simulink model "bit32cpu"  (R2020a)
settings: Solver=VariableStepAuto  StartTime=0.0  StopTime=10.0  RelTol=1e-3
libraries: simulink_extras x392
(part 17 of 63)

== system bit32cpu/ALU/Subsystem7/Subsystem3/Subsystem4/Subsystem5 ==
  In1 : Inport
  In2 : Inport  Port=2
  In3 : Inport  Port=3
  In4 : Inport  Port=4
  In5 : Inport  Port=5
  In6 : Inport  Port=6
  In7 : Inport  Port=7
  NAND : Logic  Operator=NAND  AllPortsSameDT=off  OutDataTypeStr=boolean
  NAND{1..2,4..6} (5 alike) : Logic  Operator=NAND  Inputs=4  AllPortsSameDT=off  OutDataTypeStr=boolean
  NAND3 : Logic  Operator=NAND  AllPortsSameDT=off  OutDataTypeStr=boolean
  Out1 : Outport
  wires:
  NAND6/1 -> NAND1/4
  In5/1 -> NAND5/3
  NAND3/1 -> NAND4/2, NAND2/2
  In1/1 -> NAND6/2, NAND5/2, NAND3/2, NAND3/1
  In2/1 -> NAND6/1, NAND4/1, NAND/2, NAND/1
  In4/1 -> NAND4/3
  In3/1 -> NAND2/3
  NAND/1 -> NAND5/1, NAND2/1
  NAND1/1 -> Out1/1
  In6/1 -> NAND6/3
  NAND5/1 -> NAND1/3
  NAND4/1 -> NAND1/2
  In7/1 -> NAND2/4, NAND4/4, NAND5/4, NAND6/4
  NAND2/1 -> NAND1/1

== system bit32cpu/ALU/Subsystem7/Subsystem3/Subsystem4/Subsystem6 ==
  In1 : Inport
  In2 : Inport  Port=2
  In3 : Inport  Port=3
  In4 : Inport  Port=4
  In5 : Inport  Port=5
  In6 : Inport  Port=6
  In7 : Inport  Port=7
  NAND : Logic  Operator=NAND  AllPortsSameDT=off  OutDataTypeStr=boolean
  NAND{1..2,4..6} (5 alike) : Logic  Operator=NAND  Inputs=4  AllPortsSameDT=off  OutDataTypeStr=boolean
  NAND3 : Logic  Operator=NAND  AllPortsSameDT=off  OutDataTypeStr=boolean
  Out1 : Outport
  wires:
  NAND6/1 -> NAND1/4
  In5/1 -> NAND5/3
  NAND3/1 -> NAND4/2, NAND2/2
  In1/1 -> NAND6/2, NAND5/2, NAND3/2, NAND3/1
  In2/1 -> NAND6/1, NAND4/1, NAND/2, NAND/1
  In4/1 -> NAND4/3
  In3/1 -> NAND2/3
  NAND/1 -> NAND5/1, NAND2/1
  NAND1/1 -> Out1/1
  In6/1 -> NAND6/3
  NAND5/1 -> NAND1/3
  NAND4/1 -> NAND1/2
  In7/1 -> NAND2/4, NAND4/4, NAND5/4, NAND6/4
  NAND2/1 -> NAND1/1

== system bit32cpu/ALU/Subsystem7/Subsystem3/Subsystem4/Subsystem7 ==
  In1 : Inport
  In2 : Inport  Port=2
  In3 : Inport  Port=3
  In4 : Inport  Port=4
  In5 : Inport  Port=5
  In6 : Inport  Port=6
  In7 : Inport  Port=7
  NAND : Logic  Operator=NAND  AllPortsSameDT=off  OutDataTypeStr=boolean
  NAND{1..2,4..6} (5 alike) : Logic  Operator=NAND  Inputs=4  AllPortsSameDT=off  OutDataTypeStr=boolean
  NAND3 : Logic  Operator=NAND  AllPortsSameDT=off  OutDataTypeStr=boolean
  Out1 : Outport
  wires:
  NAND6/1 -> NAND1/4
  In5/1 -> NAND5/3
  NAND3/1 -> NAND4/2, NAND2/2
  In1/1 -> NAND6/2, NAND5/2, NAND3/2, NAND3/1
  In2/1 -> NAND6/1, NAND4/1, NAND/2, NAND/1
  In4/1 -> NAND4/3
  In3/1 -> NAND2/3
  NAND/1 -> NAND5/1, NAND2/1
  NAND1/1 -> Out1/1
  In6/1 -> NAND6/3
  NAND5/1 -> NAND1/3
  NAND4/1 -> NAND1/2
  In7/1 -> NAND2/4, NAND4/4, NAND5/4, NAND6/4
  NAND2/1 -> NAND1/1

== system bit32cpu/ALU/Subsystem7/Subsystem3/Subsystem5/Subsystem ==
  In1 : Inport
  In2 : Inport  Port=2
  In3 : Inport  Port=3
  In4 : Inport  Port=4
  In5 : Inport  Port=5
  In6 : Inport  Port=6
  In7 : Inport  Port=7
  NAND : Logic  Operator=NAND  AllPortsSameDT=off  OutDataTypeStr=boolean
  NAND{1..2,4..6} (5 alike) : Logic  Operator=NAND  Inputs=4  AllPortsSameDT=off  OutDataTypeStr=boolean
  NAND3 : Logic  Operator=NAND  AllPortsSameDT=off  OutDataTypeStr=boolean
  Out1 : Outport
  wires:
  NAND6/1 -> NAND1/4
  In5/1 -> NAND5/3
  NAND3/1 -> NAND4/2, NAND2/2
  In1/1 -> NAND6/2, NAND5/2, NAND3/2, NAND3/1
  In2/1 -> NAND6/1, NAND4/1, NAND/2, NAND/1
  In4/1 -> NAND4/3
  In3/1 -> NAND2/3
  NAND/1 -> NAND5/1, NAND2/1
  NAND1/1 -> Out1/1
  In6/1 -> NAND6/3
  NAND5/1 -> NAND1/3
  NAND4/1 -> NAND1/2
  In7/1 -> NAND2/4, NAND4/4, NAND5/4, NAND6/4
  NAND2/1 -> NAND1/1

== system bit32cpu/ALU/Subsystem7/Subsystem3/Subsystem5/Subsystem1 ==
  In1 : Inport
  In2 : Inport  Port=2
  In3 : Inport  Port=3
  In4 : Inport  Port=4
  In5 : Inport  Port=5
  In6 : Inport  Port=6
  In7 : Inport  Port=7
  NAND : Logic  Operator=NAND  AllPortsSameDT=off  OutDataTypeStr=boolean
  NAND{1..2,4..6} (5 alike) : Logic  Operator=NAND  Inputs=4  AllPortsSameDT=off  OutDataTypeStr=boolean
  NAND3 : Logic  Operator=NAND  AllPortsSameDT=off  OutDataTypeStr=boolean
  Out1 : Outport
  wires:
  NAND6/1 -> NAND1/4
  In5/1 -> NAND5/3
  NAND3/1 -> NAND4/2, NAND2/2
  In1/1 -> NAND6/2, NAND5/2, NAND3/2, NAND3/1
  In2/1 -> NAND6/1, NAND4/1, NAND/2, NAND/1
  In4/1 -> NAND4/3
  In3/1 -> NAND2/3
  NAND/1 -> NAND5/1, NAND2/1
  NAND1/1 -> Out1/1
  In6/1 -> NAND6/3
  NAND5/1 -> NAND1/3
  NAND4/1 -> NAND1/2
  In7/1 -> NAND2/4, NAND4/4, NAND5/4, NAND6/4
  NAND2/1 -> NAND1/1

== system bit32cpu/ALU/Subsystem7/Subsystem3/Subsystem5/Subsystem2 ==
  In1 : Inport
  In2 : Inport  Port=2
  In3 : Inport  Port=3
  In4 : Inport  Port=4
  In5 : Inport  Port=5
  In6 : Inport  Port=6
  In7 : Inport  Port=7
  NAND : Logic  Operator=NAND  AllPortsSameDT=off  OutDataTypeStr=boolean
  NAND{1..2,4..6} (5 alike) : Logic  Operator=NAND  Inputs=4  AllPortsSameDT=off  OutDataTypeStr=boolean
  NAND3 : Logic  Operator=NAND  AllPortsSameDT=off  OutDataTypeStr=boolean
  Out1 : Outport
  wires:
  NAND6/1 -> NAND1/4
  In5/1 -> NAND5/3
  NAND3/1 -> NAND4/2, NAND2/2
  In1/1 -> NAND6/2, NAND5/2, NAND3/2, NAND3/1
  In2/1 -> NAND6/1, NAND4/1, NAND/2, NAND/1
  In4/1 -> NAND4/3
  In3/1 -> NAND2/3
  NAND/1 -> NAND5/1, NAND2/1
  NAND1/1 -> Out1/1
  In6/1 -> NAND6/3
  NAND5/1 -> NAND1/3
  NAND4/1 -> NAND1/2
  In7/1 -> NAND2/4, NAND4/4, NAND5/4, NAND6/4
  NAND2/1 -> NAND1/1

== system bit32cpu/ALU/Subsystem7/Subsystem3/Subsystem5/Subsystem3 ==
  In1 : Inport
  In2 : Inport  Port=2
  In3 : Inport  Port=3
  In4 : Inport  Port=4
  In5 : Inport  Port=5
  In6 : Inport  Port=6
  In7 : Inport  Port=7
  NAND : Logic  Operator=NAND  AllPortsSameDT=off  OutDataTypeStr=boolean
  NAND{1..2,4..6} (5 alike) : Logic  Operator=NAND  Inputs=4  AllPortsSameDT=off  OutDataTypeStr=boolean
  NAND3 : Logic  Operator=NAND  AllPortsSameDT=off  OutDataTypeStr=boolean
  Out1 : Outport
  wires:
  NAND6/1 -> NAND1/4
  In5/1 -> NAND5/3
  NAND3/1 -> NAND4/2, NAND2/2
  In1/1 -> NAND6/2, NAND5/2, NAND3/2, NAND3/1
  In2/1 -> NAND6/1, NAND4/1, NAND/2, NAND/1
  In4/1 -> NAND4/3
  In3/1 -> NAND2/3
  NAND/1 -> NAND5/1, NAND2/1
  NAND1/1 -> Out1/1
  In6/1 -> NAND6/3
  NAND5/1 -> NAND1/3
  NAND4/1 -> NAND1/2
  In7/1 -> NAND2/4, NAND4/4, NAND5/4, NAND6/4
  NAND2/1 -> NAND1/1

== system bit32cpu/ALU/Subsystem7/Subsystem3/Subsystem5/Subsystem4 ==
  In1 : Inport
  In2 : Inport  Port=2
  In3 : Inport  Port=3
  In4 : Inport  Port=4
  In5 : Inport  Port=5
  In6 : Inport  Port=6
  In7 : Inport  Port=7
  NAND : Logic  Operator=NAND  AllPortsSameDT=off  OutDataTypeStr=boolean
  NAND{1..2,4..6} (5 alike) : Logic  Operator=NAND  Inputs=4  AllPortsSameDT=off  OutDataTypeStr=boolean
  NAND3 : Logic  Operator=NAND  AllPortsSameDT=off  OutDataTypeStr=boolean
  Out1 : Outport
  wires:
  NAND6/1 -> NAND1/4
  In5/1 -> NAND5/3
  NAND3/1 -> NAND4/2, NAND2/2
  In1/1 -> NAND6/2, NAND5/2, NAND3/2, NAND3/1
  In2/1 -> NAND6/1, NAND4/1, NAND/2, NAND/1
  In4/1 -> NAND4/3
  In3/1 -> NAND2/3
  NAND/1 -> NAND5/1, NAND2/1
  NAND1/1 -> Out1/1
  In6/1 -> NAND6/3
  NAND5/1 -> NAND1/3
  NAND4/1 -> NAND1/2
  In7/1 -> NAND2/4, NAND4/4, NAND5/4, NAND6/4
  NAND2/1 -> NAND1/1

== system bit32cpu/ALU/Subsystem7/Subsystem3/Subsystem5/Subsystem5 ==
  In1 : Inport
  In2 : Inport  Port=2
  In3 : Inport  Port=3
  In4 : Inport  Port=4
  In5 : Inport  Port=5
  In6 : Inport  Port=6
  In7 : Inport  Port=7
  NAND : Logic  Operator=NAND  AllPortsSameDT=off  OutDataTypeStr=boolean
  NAND{1..2,4..6} (5 alike) : Logic  Operator=NAND  Inputs=4  AllPortsSameDT=off  OutDataTypeStr=boolean
  NAND3 : Logic  Operator=NAND  AllPortsSameDT=off  OutDataTypeStr=boolean
  Out1 : Outport
  wires:
  NAND6/1 -> NAND1/4
  In5/1 -> NAND5/3
  NAND3/1 -> NAND4/2, NAND2/2
  In1/1 -> NAND6/2, NAND5/2, NAND3/2, NAND3/1
  In2/1 -> NAND6/1, NAND4/1, NAND/2, NAND/1
  In4/1 -> NAND4/3
  In3/1 -> NAND2/3
  NAND/1 -> NAND5/1, NAND2/1
  NAND1/1 -> Out1/1
  In6/1 -> NAND6/3
  NAND5/1 -> NAND1/3
  NAND4/1 -> NAND1/2
  In7/1 -> NAND2/4, NAND4/4, NAND5/4, NAND6/4
  NAND2/1 -> NAND1/1

== system bit32cpu/ALU/Subsystem7/Subsystem3/Subsystem5/Subsystem6 ==
  In1 : Inport
  In2 : Inport  Port=2
  In3 : Inport  Port=3
  In4 : Inport  Port=4
  In5 : Inport  Port=5
  In6 : Inport  Port=6
  In7 : Inport  Port=7
  NAND : Logic  Operator=NAND  AllPortsSameDT=off  OutDataTypeStr=boolean
  NAND{1..2,4..6} (5 alike) : Logic  Operator=NAND  Inputs=4  AllPortsSameDT=off  OutDataTypeStr=boolean
  NAND3 : Logic  Operator=NAND  AllPortsSameDT=off  OutDataTypeStr=boolean
  Out1 : Outport
  wires:
  NAND6/1 -> NAND1/4
  In5/1 -> NAND5/3
  NAND3/1 -> NAND4/2, NAND2/2
  In1/1 -> NAND6/2, NAND5/2, NAND3/2, NAND3/1
  In2/1 -> NAND6/1, NAND4/1, NAND/2, NAND/1
  In4/1 -> NAND4/3
  In3/1 -> NAND2/3
  NAND/1 -> NAND5/1, NAND2/1
  NAND1/1 -> Out1/1
  In6/1 -> NAND6/3
  NAND5/1 -> NAND1/3
  NAND4/1 -> NAND1/2
  In7/1 -> NAND2/4, NAND4/4, NAND5/4, NAND6/4
  NAND2/1 -> NAND1/1

== system bit32cpu/ALU/Subsystem7/Subsystem3/Subsystem5/Subsystem7 ==
  In1 : Inport
  In2 : Inport  Port=2
  In3 : Inport  Port=3
  In4 : Inport  Port=4
  In5 : Inport  Port=5
  In6 : Inport  Port=6
  In7 : Inport  Port=7
  NAND : Logic  Operator=NAND  AllPortsSameDT=off  OutDataTypeStr=boolean
  NAND{1..2,4..6} (5 alike) : Logic  Operator=NAND  Inputs=4  AllPortsSameDT=off  OutDataTypeStr=boolean
  NAND3 : Logic  Operator=NAND  AllPortsSameDT=off  OutDataTypeStr=boolean
  Out1 : Outport
  wires:
  NAND6/1 -> NAND1/4
  In5/1 -> NAND5/3
  NAND3/1 -> NAND4/2, NAND2/2
  In1/1 -> NAND6/2, NAND5/2, NAND3/2, NAND3/1
  In2/1 -> NAND6/1, NAND4/1, NAND/2, NAND/1
  In4/1 -> NAND4/3
  In3/1 -> NAND2/3
  NAND/1 -> NAND5/1, NAND2/1
  NAND1/1 -> Out1/1
  In6/1 -> NAND6/3
  NAND5/1 -> NAND1/3
  NAND4/1 -> NAND1/2
  In7/1 -> NAND2/4, NAND4/4, NAND5/4, NAND6/4
  NAND2/1 -> NAND1/1

== system bit32cpu/ALU/Subsystem7/Subsystem4/Subsystem1/Subsystem ==
  In1 : Inport
  In2 : Inport  Port=2
  In3 : Inport  Port=3
  In4 : Inport  Port=4
  In5 : Inport  Port=5
  In6 : Inport  Port=6
  In7 : Inport  Port=7
  NAND : Logic  Operator=NAND  AllPortsSameDT=off  OutDataTypeStr=boolean
  NAND{1..2,4..6} (5 alike) : Logic  Operator=NAND  Inputs=4  AllPortsSameDT=off  OutDataTypeStr=boolean
  NAND3 : Logic  Operator=NAND  AllPortsSameDT=off  OutDataTypeStr=boolean
  Out1 : Outport
  wires:
  NAND6/1 -> NAND1/4
  In5/1 -> NAND5/3
  NAND3/1 -> NAND4/2, NAND2/2
  In1/1 -> NAND6/2, NAND5/2, NAND3/2, NAND3/1
  In2/1 -> NAND6/1, NAND4/1, NAND/2, NAND/1
  In4/1 -> NAND4/3
  In3/1 -> NAND2/3
  NAND/1 -> NAND5/1, NAND2/1
  NAND1/1 -> Out1/1
  In6/1 -> NAND6/3
  NAND5/1 -> NAND1/3
  NAND4/1 -> NAND1/2
  In7/1 -> NAND2/4, NAND4/4, NAND5/4, NAND6/4
  NAND2/1 -> NAND1/1

== system bit32cpu/ALU/Subsystem7/Subsystem4/Subsystem1/Subsystem1 ==
  In1 : Inport
  In2 : Inport  Port=2
  In3 : Inport  Port=3
  In4 : Inport  Port=4
  In5 : Inport  Port=5
  In6 : Inport  Port=6
  In7 : Inport  Port=7
  NAND : Logic  Operator=NAND  AllPortsSameDT=off  OutDataTypeStr=boolean
  NAND{1..2,4..6} (5 alike) : Logic  Operator=NAND  Inputs=4  AllPortsSameDT=off  OutDataTypeStr=boolean
  NAND3 : Logic  Operator=NAND  AllPortsSameDT=off  OutDataTypeStr=boolean
  Out1 : Outport
  wires:
  NAND6/1 -> NAND1/4
  In5/1 -> NAND5/3
  NAND3/1 -> NAND4/2, NAND2/2
  In1/1 -> NAND6/2, NAND5/2, NAND3/2, NAND3/1
  In2/1 -> NAND6/1, NAND4/1, NAND/2, NAND/1
  In4/1 -> NAND4/3
  In3/1 -> NAND2/3
  NAND/1 -> NAND5/1, NAND2/1
  NAND1/1 -> Out1/1
  In6/1 -> NAND6/3
  NAND5/1 -> NAND1/3
  NAND4/1 -> NAND1/2
  In7/1 -> NAND2/4, NAND4/4, NAND5/4, NAND6/4
  NAND2/1 -> NAND1/1

== system bit32cpu/ALU/Subsystem7/Subsystem4/Subsystem1/Subsystem2 ==
  In1 : Inport
  In2 : Inport  Port=2
  In3 : Inport  Port=3
  In4 : Inport  Port=4
  In5 : Inport  Port=5
  In6 : Inport  Port=6
  In7 : Inport  Port=7
  NAND : Logic  Operator=NAND  AllPortsSameDT=off  OutDataTypeStr=boolean
  NAND{1..2,4..6} (5 alike) : Logic  Operator=NAND  Inputs=4  AllPortsSameDT=off  OutDataTypeStr=boolean
  NAND3 : Logic  Operator=NAND  AllPortsSameDT=off  OutDataTypeStr=boolean
  Out1 : Outport
  wires:
  NAND6/1 -> NAND1/4
  In5/1 -> NAND5/3
  NAND3/1 -> NAND4/2, NAND2/2
  In1/1 -> NAND6/2, NAND5/2, NAND3/2, NAND3/1
  In2/1 -> NAND6/1, NAND4/1, NAND/2, NAND/1
  In4/1 -> NAND4/3
  In3/1 -> NAND2/3
  NAND/1 -> NAND5/1, NAND2/1
  NAND1/1 -> Out1/1
  In6/1 -> NAND6/3
  NAND5/1 -> NAND1/3
  NAND4/1 -> NAND1/2
  In7/1 -> NAND2/4, NAND4/4, NAND5/4, NAND6/4
  NAND2/1 -> NAND1/1

== system bit32cpu/ALU/Subsystem7/Subsystem4/Subsystem1/Subsystem3 ==
  In1 : Inport
  In2 : Inport  Port=2
  In3 : Inport  Port=3
  In4 : Inport  Port=4
  In5 : Inport  Port=5
  In6 : Inport  Port=6
  In7 : Inport  Port=7
  NAND : Logic  Operator=NAND  AllPortsSameDT=off  OutDataTypeStr=boolean
  NAND{1..2,4..6} (5 alike) : Logic  Operator=NAND  Inputs=4  AllPortsSameDT=off  OutDataTypeStr=boolean
  NAND3 : Logic  Operator=NAND  AllPortsSameDT=off  OutDataTypeStr=boolean
  Out1 : Outport
  wires:
  NAND6/1 -> NAND1/4
  In5/1 -> NAND5/3
  NAND3/1 -> NAND4/2, NAND2/2
  In1/1 -> NAND6/2, NAND5/2, NAND3/2, NAND3/1
  In2/1 -> NAND6/1, NAND4/1, NAND/2, NAND/1
  In4/1 -> NAND4/3
  In3/1 -> NAND2/3
  NAND/1 -> NAND5/1, NAND2/1
  NAND1/1 -> Out1/1
  In6/1 -> NAND6/3
  NAND5/1 -> NAND1/3
  NAND4/1 -> NAND1/2
  In7/1 -> NAND2/4, NAND4/4, NAND5/4, NAND6/4
  NAND2/1 -> NAND1/1

== system bit32cpu/ALU/Subsystem7/Subsystem4/Subsystem1/Subsystem4 ==
  In1 : Inport
  In2 : Inport  Port=2
  In3 : Inport  Port=3
  In4 : Inport  Port=4
  In5 : Inport  Port=5
  In6 : Inport  Port=6
  In7 : Inport  Port=7
  NAND : Logic  Operator=NAND  AllPortsSameDT=off  OutDataTypeStr=boolean
  NAND{1..2,4..6} (5 alike) : Logic  Operator=NAND  Inputs=4  AllPortsSameDT=off  OutDataTypeStr=boolean
  NAND3 : Logic  Operator=NAND  AllPortsSameDT=off  OutDataTypeStr=boolean
  Out1 : Outport
  wires:
  NAND6/1 -> NAND1/4
  In5/1 -> NAND5/3
  NAND3/1 -> NAND4/2, NAND2/2
  In1/1 -> NAND6/2, NAND5/2, NAND3/2, NAND3/1
  In2/1 -> NAND6/1, NAND4/1, NAND/2, NAND/1
  In4/1 -> NAND4/3
  In3/1 -> NAND2/3
  NAND/1 -> NAND5/1, NAND2/1
  NAND1/1 -> Out1/1
  In6/1 -> NAND6/3
  NAND5/1 -> NAND1/3
  NAND4/1 -> NAND1/2
  In7/1 -> NAND2/4, NAND4/4, NAND5/4, NAND6/4
  NAND2/1 -> NAND1/1

== system bit32cpu/ALU/Subsystem7/Subsystem4/Subsystem1/Subsystem5 ==
  In1 : Inport
  In2 : Inport  Port=2
  In3 : Inport  Port=3
  In4 : Inport  Port=4
  In5 : Inport  Port=5
  In6 : Inport  Port=6
  In7 : Inport  Port=7
  NAND : Logic  Operator=NAND  AllPortsSameDT=off  OutDataTypeStr=boolean
  NAND{1..2,4..6} (5 alike) : Logic  Operator=NAND  Inputs=4  AllPortsSameDT=off  OutDataTypeStr=boolean
  NAND3 : Logic  Operator=NAND  AllPortsSameDT=off  OutDataTypeStr=boolean
  Out1 : Outport
  wires:
  NAND6/1 -> NAND1/4
  In5/1 -> NAND5/3
  NAND3/1 -> NAND4/2, NAND2/2
  In1/1 -> NAND6/2, NAND5/2, NAND3/2, NAND3/1
  In2/1 -> NAND6/1, NAND4/1, NAND/2, NAND/1
  In4/1 -> NAND4/3
  In3/1 -> NAND2/3
  NAND/1 -> NAND5/1, NAND2/1
  NAND1/1 -> Out1/1
  In6/1 -> NAND6/3
  NAND5/1 -> NAND1/3
  NAND4/1 -> NAND1/2
  In7/1 -> NAND2/4, NAND4/4, NAND5/4, NAND6/4
  NAND2/1 -> NAND1/1

== system bit32cpu/ALU/Subsystem7/Subsystem4/Subsystem1/Subsystem6 ==
  In1 : Inport
  In2 : Inport  Port=2
  In3 : Inport  Port=3
  In4 : Inport  Port=4
  In5 : Inport  Port=5
  In6 : Inport  Port=6
  In7 : Inport  Port=7
  NAND : Logic  Operator=NAND  AllPortsSameDT=off  OutDataTypeStr=boolean
  NAND{1..2,4..6} (5 alike) : Logic  Operator=NAND  Inputs=4  AllPortsSameDT=off  OutDataTypeStr=boolean
  NAND3 : Logic  Operator=NAND  AllPortsSameDT=off  OutDataTypeStr=boolean
  Out1 : Outport
  wires:
  NAND6/1 -> NAND1/4
  In5/1 -> NAND5/3
  NAND3/1 -> NAND4/2, NAND2/2
  In1/1 -> NAND6/2, NAND5/2, NAND3/2, NAND3/1
  In2/1 -> NAND6/1, NAND4/1, NAND/2, NAND/1
  In4/1 -> NAND4/3
  In3/1 -> NAND2/3
  NAND/1 -> NAND5/1, NAND2/1
  NAND1/1 -> Out1/1
  In6/1 -> NAND6/3
  NAND5/1 -> NAND1/3
  NAND4/1 -> NAND1/2
  In7/1 -> NAND2/4, NAND4/4, NAND5/4, NAND6/4
  NAND2/1 -> NAND1/1

== system bit32cpu/ALU/Subsystem7/Subsystem4/Subsystem1/Subsystem7 ==
  In1 : Inport
  In2 : Inport  Port=2
  In3 : Inport  Port=3
  In4 : Inport  Port=4
  In5 : Inport  Port=5
  In6 : Inport  Port=6
  In7 : Inport  Port=7
  NAND : Logic  Operator=NAND  AllPortsSameDT=off  OutDataTypeStr=boolean
  NAND{1..2,4..6} (5 alike) : Logic  Operator=NAND  Inputs=4  AllPortsSameDT=off  OutDataTypeStr=boolean
  NAND3 : Logic  Operator=NAND  AllPortsSameDT=off  OutDataTypeStr=boolean
  Out1 : Outport
  wires:
  NAND6/1 -> NAND1/4
  In5/1 -> NAND5/3
  NAND3/1 -> NAND4/2, NAND2/2
  In1/1 -> NAND6/2, NAND5/2, NAND3/2, NAND3/1
  In2/1 -> NAND6/1, NAND4/1, NAND/2, NAND/1
  In4/1 -> NAND4/3
  In3/1 -> NAND2/3
  NAND/1 -> NAND5/1, NAND2/1
  NAND1/1 -> Out1/1
  In6/1 -> NAND6/3
  NAND5/1 -> NAND1/3
  NAND4/1 -> NAND1/2
  In7/1 -> NAND2/4, NAND4/4, NAND5/4, NAND6/4
  NAND2/1 -> NAND1/1

== system bit32cpu/ALU/Subsystem7/Subsystem4/Subsystem2/Subsystem ==
  In1 : Inport
  In2 : Inport  Port=2
  In3 : Inport  Port=3
  In4 : Inport  Port=4
  In5 : Inport  Port=5
  In6 : Inport  Port=6
  In7 : Inport  Port=7
  NAND : Logic  Operator=NAND  AllPortsSameDT=off  OutDataTypeStr=boolean
  NAND{1..2,4..6} (5 alike) : Logic  Operator=NAND  Inputs=4  AllPortsSameDT=off  OutDataTypeStr=boolean
  NAND3 : Logic  Operator=NAND  AllPortsSameDT=off  OutDataTypeStr=boolean
  Out1 : Outport
  wires:
  NAND6/1 -> NAND1/4
  In5/1 -> NAND5/3
  NAND3/1 -> NAND4/2, NAND2/2
  In1/1 -> NAND6/2, NAND5/2, NAND3/2, NAND3/1
  In2/1 -> NAND6/1, NAND4/1, NAND/2, NAND/1
  In4/1 -> NAND4/3
  In3/1 -> NAND2/3
  NAND/1 -> NAND5/1, NAND2/1
  NAND1/1 -> Out1/1
  In6/1 -> NAND6/3
  NAND5/1 -> NAND1/3
  NAND4/1 -> NAND1/2
  In7/1 -> NAND2/4, NAND4/4, NAND5/4, NAND6/4
  NAND2/1 -> NAND1/1

== system bit32cpu/ALU/Subsystem7/Subsystem4/Subsystem2/Subsystem1 ==
  In1 : Inport
  In2 : Inport  Port=2
  In3 : Inport  Port=3
  In4 : Inport  Port=4
  In5 : Inport  Port=5
  In6 : Inport  Port=6
  In7 : Inport  Port=7
  NAND : Logic  Operator=NAND  AllPortsSameDT=off  OutDataTypeStr=boolean
  NAND{1..2,4..6} (5 alike) : Logic  Operator=NAND  Inputs=4  AllPortsSameDT=off  OutDataTypeStr=boolean
  NAND3 : Logic  Operator=NAND  AllPortsSameDT=off  OutDataTypeStr=boolean
  Out1 : Outport
  wires:
  NAND6/1 -> NAND1/4
  In5/1 -> NAND5/3
  NAND3/1 -> NAND4/2, NAND2/2
  In1/1 -> NAND6/2, NAND5/2, NAND3/2, NAND3/1
  In2/1 -> NAND6/1, NAND4/1, NAND/2, NAND/1
  In4/1 -> NAND4/3
  In3/1 -> NAND2/3
  NAND/1 -> NAND5/1, NAND2/1
  NAND1/1 -> Out1/1
  In6/1 -> NAND6/3
  NAND5/1 -> NAND1/3
  NAND4/1 -> NAND1/2
  In7/1 -> NAND2/4, NAND4/4, NAND5/4, NAND6/4
  NAND2/1 -> NAND1/1

== system bit32cpu/ALU/Subsystem7/Subsystem4/Subsystem2/Subsystem2 ==
  In1 : Inport
  In2 : Inport  Port=2
  In3 : Inport  Port=3
  In4 : Inport  Port=4
  In5 : Inport  Port=5
  In6 : Inport  Port=6
  In7 : Inport  Port=7
  NAND : Logic  Operator=NAND  AllPortsSameDT=off  OutDataTypeStr=boolean
  NAND{1..2,4..6} (5 alike) : Logic  Operator=NAND  Inputs=4  AllPortsSameDT=off  OutDataTypeStr=boolean
  NAND3 : Logic  Operator=NAND  AllPortsSameDT=off  OutDataTypeStr=boolean
  Out1 : Outport
  wires:
  NAND6/1 -> NAND1/4
  In5/1 -> NAND5/3
  NAND3/1 -> NAND4/2, NAND2/2
  In1/1 -> NAND6/2, NAND5/2, NAND3/2, NAND3/1
  In2/1 -> NAND6/1, NAND4/1, NAND/2, NAND/1
  In4/1 -> NAND4/3
  In3/1 -> NAND2/3
  NAND/1 -> NAND5/1, NAND2/1
  NAND1/1 -> Out1/1
  In6/1 -> NAND6/3
  NAND5/1 -> NAND1/3
  NAND4/1 -> NAND1/2
  In7/1 -> NAND2/4, NAND4/4, NAND5/4, NAND6/4
  NAND2/1 -> NAND1/1

== system bit32cpu/ALU/Subsystem7/Subsystem4/Subsystem2/Subsystem3 ==
  In1 : Inport
  In2 : Inport  Port=2
  In3 : Inport  Port=3
  In4 : Inport  Port=4
  In5 : Inport  Port=5
  In6 : Inport  Port=6
  In7 : Inport  Port=7
  NAND : Logic  Operator=NAND  AllPortsSameDT=off  OutDataTypeStr=boolean
  NAND{1..2,4..6} (5 alike) : Logic  Operator=NAND  Inputs=4  AllPortsSameDT=off  OutDataTypeStr=boolean
  NAND3 : Logic  Operator=NAND  AllPortsSameDT=off  OutDataTypeStr=boolean
  Out1 : Outport
  wires:
  NAND6/1 -> NAND1/4
  In5/1 -> NAND5/3
  NAND3/1 -> NAND4/2, NAND2/2
  In1/1 -> NAND6/2, NAND5/2, NAND3/2, NAND3/1
  In2/1 -> NAND6/1, NAND4/1, NAND/2, NAND/1
  In4/1 -> NAND4/3
  In3/1 -> NAND2/3
  NAND/1 -> NAND5/1, NAND2/1
  NAND1/1 -> Out1/1
  In6/1 -> NAND6/3
  NAND5/1 -> NAND1/3
  NAND4/1 -> NAND1/2
  In7/1 -> NAND2/4, NAND4/4, NAND5/4, NAND6/4
  NAND2/1 -> NAND1/1

== system bit32cpu/ALU/Subsystem7/Subsystem4/Subsystem2/Subsystem4 ==
  In1 : Inport
  In2 : Inport  Port=2
  In3 : Inport  Port=3
  In4 : Inport  Port=4
  In5 : Inport  Port=5
  In6 : Inport  Port=6
  In7 : Inport  Port=7
  NAND : Logic  Operator=NAND  AllPortsSameDT=off  OutDataTypeStr=boolean
  NAND{1..2,4..6} (5 alike) : Logic  Operator=NAND  Inputs=4  AllPortsSameDT=off  OutDataTypeStr=boolean
  NAND3 : Logic  Operator=NAND  AllPortsSameDT=off  OutDataTypeStr=boolean
  Out1 : Outport
  wires:
  NAND6/1 -> NAND1/4
  In5/1 -> NAND5/3
  NAND3/1 -> NAND4/2, NAND2/2
  In1/1 -> NAND6/2, NAND5/2, NAND3/2, NAND3/1
  In2/1 -> NAND6/1, NAND4/1, NAND/2, NAND/1
  In4/1 -> NAND4/3
  In3/1 -> NAND2/3
  NAND/1 -> NAND5/1, NAND2/1
  NAND1/1 -> Out1/1
  In6/1 -> NAND6/3
  NAND5/1 -> NAND1/3
  NAND4/1 -> NAND1/2
  In7/1 -> NAND2/4, NAND4/4, NAND5/4, NAND6/4
  NAND2/1 -> NAND1/1

== system bit32cpu/ALU/Subsystem7/Subsystem4/Subsystem2/Subsystem5 ==
  In1 : Inport
  In2 : Inport  Port=2
  In3 : Inport  Port=3
  In4 : Inport  Port=4
  In5 : Inport  Port=5
  In6 : Inport  Port=6
  In7 : Inport  Port=7
  NAND : Logic  Operator=NAND  AllPortsSameDT=off  OutDataTypeStr=boolean
  NAND{1..2,4..6} (5 alike) : Logic  Operator=NAND  Inputs=4  AllPortsSameDT=off  OutDataTypeStr=boolean
  NAND3 : Logic  Operator=NAND  AllPortsSameDT=off  OutDataTypeStr=boolean
  Out1 : Outport
  wires:
  NAND6/1 -> NAND1/4
  In5/1 -> NAND5/3
  NAND3/1 -> NAND4/2, NAND2/2
  In1/1 -> NAND6/2, NAND5/2, NAND3/2, NAND3/1
  In2/1 -> NAND6/1, NAND4/1, NAND/2, NAND/1
  In4/1 -> NAND4/3
  In3/1 -> NAND2/3
  NAND/1 -> NAND5/1, NAND2/1
  NAND1/1 -> Out1/1
  In6/1 -> NAND6/3
  NAND5/1 -> NAND1/3
  NAND4/1 -> NAND1/2
  In7/1 -> NAND2/4, NAND4/4, NAND5/4, NAND6/4
  NAND2/1 -> NAND1/1

== system bit32cpu/ALU/Subsystem7/Subsystem4/Subsystem2/Subsystem6 ==
  In1 : Inport
  In2 : Inport  Port=2
  In3 : Inport  Port=3
  In4 : Inport  Port=4
  In5 : Inport  Port=5
  In6 : Inport  Port=6
  In7 : Inport  Port=7
  NAND : Logic  Operator=NAND  AllPortsSameDT=off  OutDataTypeStr=boolean
  NAND{1..2,4..6} (5 alike) : Logic  Operator=NAND  Inputs=4  AllPortsSameDT=off  OutDataTypeStr=boolean
  NAND3 : Logic  Operator=NAND  AllPortsSameDT=off  OutDataTypeStr=boolean
  Out1 : Outport
  wires:
  NAND6/1 -> NAND1/4
  In5/1 -> NAND5/3
  NAND3/1 -> NAND4/2, NAND2/2
  In1/1 -> NAND6/2, NAND5/2, NAND3/2, NAND3/1
  In2/1 -> NAND6/1, NAND4/1, NAND/2, NAND/1
  In4/1 -> NAND4/3
  In3/1 -> NAND2/3
  NAND/1 -> NAND5/1, NAND2/1
  NAND1/1 -> Out1/1
  In6/1 -> NAND6/3
  NAND5/1 -> NAND1/3
  NAND4/1 -> NAND1/2
  In7/1 -> NAND2/4, NAND4/4, NAND5/4, NAND6/4
  NAND2/1 -> NAND1/1

== system bit32cpu/ALU/Subsystem7/Subsystem4/Subsystem2/Subsystem7 ==
  In1 : Inport
  In2 : Inport  Port=2
  In3 : Inport  Port=3
  In4 : Inport  Port=4
  In5 : Inport  Port=5
  In6 : Inport  Port=6
  In7 : Inport  Port=7
  NAND : Logic  Operator=NAND  AllPortsSameDT=off  OutDataTypeStr=boolean
  NAND{1..2,4..6} (5 alike) : Logic  Operator=NAND  Inputs=4  AllPortsSameDT=off  OutDataTypeStr=boolean
  NAND3 : Logic  Operator=NAND  AllPortsSameDT=off  OutDataTypeStr=boolean
  Out1 : Outport
  wires:
  NAND6/1 -> NAND1/4
  In5/1 -> NAND5/3
  NAND3/1 -> NAND4/2, NAND2/2
  In1/1 -> NAND6/2, NAND5/2, NAND3/2, NAND3/1
  In2/1 -> NAND6/1, NAND4/1, NAND/2, NAND/1
  In4/1 -> NAND4/3
  In3/1 -> NAND2/3
  NAND/1 -> NAND5/1, NAND2/1
  NAND1/1 -> Out1/1
  In6/1 -> NAND6/3
  NAND5/1 -> NAND1/3
  NAND4/1 -> NAND1/2
  In7/1 -> NAND2/4, NAND4/4, NAND5/4, NAND6/4
  NAND2/1 -> NAND1/1

== system bit32cpu/ALU/Subsystem7/Subsystem4/Subsystem3/Subsystem ==
  In1 : Inport
  In2 : Inport  Port=2
  In3 : Inport  Port=3
  In4 : Inport  Port=4
  In5 : Inport  Port=5
  In6 : Inport  Port=6
  In7 : Inport  Port=7
  NAND : Logic  Operator=NAND  AllPortsSameDT=off  OutDataTypeStr=boolean
  NAND{1..2,4..6} (5 alike) : Logic  Operator=NAND  Inputs=4  AllPortsSameDT=off  OutDataTypeStr=boolean
  NAND3 : Logic  Operator=NAND  AllPortsSameDT=off  OutDataTypeStr=boolean
  Out1 : Outport
  wires:
  NAND6/1 -> NAND1/4
  In5/1 -> NAND5/3
  NAND3/1 -> NAND4/2, NAND2/2
  In1/1 -> NAND6/2, NAND5/2, NAND3/2, NAND3/1
  In2/1 -> NAND6/1, NAND4/1, NAND/2, NAND/1
  In4/1 -> NAND4/3
  In3/1 -> NAND2/3
  NAND/1 -> NAND5/1, NAND2/1
  NAND1/1 -> Out1/1
  In6/1 -> NAND6/3
  NAND5/1 -> NAND1/3
  NAND4/1 -> NAND1/2
  In7/1 -> NAND2/4, NAND4/4, NAND5/4, NAND6/4
  NAND2/1 -> NAND1/1

== system bit32cpu/ALU/Subsystem7/Subsystem4/Subsystem3/Subsystem1 ==
  In1 : Inport
  In2 : Inport  Port=2
  In3 : Inport  Port=3
  In4 : Inport  Port=4
  In5 : Inport  Port=5
  In6 : Inport  Port=6
  In7 : Inport  Port=7
  NAND : Logic  Operator=NAND  AllPortsSameDT=off  OutDataTypeStr=boolean
  NAND{1..2,4..6} (5 alike) : Logic  Operator=NAND  Inputs=4  AllPortsSameDT=off  OutDataTypeStr=boolean
  NAND3 : Logic  Operator=NAND  AllPortsSameDT=off  OutDataTypeStr=boolean
  Out1 : Outport
  wires:
  NAND6/1 -> NAND1/4
  In5/1 -> NAND5/3
  NAND3/1 -> NAND4/2, NAND2/2
  In1/1 -> NAND6/2, NAND5/2, NAND3/2, NAND3/1
  In2/1 -> NAND6/1, NAND4/1, NAND/2, NAND/1
  In4/1 -> NAND4/3
  In3/1 -> NAND2/3
  NAND/1 -> NAND5/1, NAND2/1
  NAND1/1 -> Out1/1
  In6/1 -> NAND6/3
  NAND5/1 -> NAND1/3
  NAND4/1 -> NAND1/2
  In7/1 -> NAND2/4, NAND4/4, NAND5/4, NAND6/4
  NAND2/1 -> NAND1/1

== system bit32cpu/ALU/Subsystem7/Subsystem4/Subsystem3/Subsystem2 ==
  In1 : Inport
  In2 : Inport  Port=2
  In3 : Inport  Port=3
  In4 : Inport  Port=4
  In5 : Inport  Port=5
  In6 : Inport  Port=6
  In7 : Inport  Port=7
  NAND : Logic  Operator=NAND  AllPortsSameDT=off  OutDataTypeStr=boolean
  NAND{1..2,4..6} (5 alike) : Logic  Operator=NAND  Inputs=4  AllPortsSameDT=off  OutDataTypeStr=boolean
  NAND3 : Logic  Operator=NAND  AllPortsSameDT=off  OutDataTypeStr=boolean
  Out1 : Outport
  wires:
  NAND6/1 -> NAND1/4
  In5/1 -> NAND5/3
  NAND3/1 -> NAND4/2, NAND2/2
  In1/1 -> NAND6/2, NAND5/2, NAND3/2, NAND3/1
  In2/1 -> NAND6/1, NAND4/1, NAND/2, NAND/1
  In4/1 -> NAND4/3
  In3/1 -> NAND2/3
  NAND/1 -> NAND5/1, NAND2/1
  NAND1/1 -> Out1/1
  In6/1 -> NAND6/3
  NAND5/1 -> NAND1/3
  NAND4/1 -> NAND1/2
  In7/1 -> NAND2/4, NAND4/4, NAND5/4, NAND6/4
  NAND2/1 -> NAND1/1

== system bit32cpu/ALU/Subsystem7/Subsystem4/Subsystem3/Subsystem3 ==
  In1 : Inport
  In2 : Inport  Port=2
  In3 : Inport  Port=3
  In4 : Inport  Port=4
  In5 : Inport  Port=5
  In6 : Inport  Port=6
  In7 : Inport  Port=7
  NAND : Logic  Operator=NAND  AllPortsSameDT=off  OutDataTypeStr=boolean
  NAND{1..2,4..6} (5 alike) : Logic  Operator=NAND  Inputs=4  AllPortsSameDT=off  OutDataTypeStr=boolean
  NAND3 : Logic  Operator=NAND  AllPortsSameDT=off  OutDataTypeStr=boolean
  Out1 : Outport
  wires:
  NAND6/1 -> NAND1/4
  In5/1 -> NAND5/3
  NAND3/1 -> NAND4/2, NAND2/2
  In1/1 -> NAND6/2, NAND5/2, NAND3/2, NAND3/1
  In2/1 -> NAND6/1, NAND4/1, NAND/2, NAND/1
  In4/1 -> NAND4/3
  In3/1 -> NAND2/3
  NAND/1 -> NAND5/1, NAND2/1
  NAND1/1 -> Out1/1
  In6/1 -> NAND6/3
  NAND5/1 -> NAND1/3
  NAND4/1 -> NAND1/2
  In7/1 -> NAND2/4, NAND4/4, NAND5/4, NAND6/4
  NAND2/1 -> NAND1/1

== system bit32cpu/ALU/Subsystem7/Subsystem4/Subsystem3/Subsystem4 ==
  In1 : Inport
  In2 : Inport  Port=2
  In3 : Inport  Port=3
  In4 : Inport  Port=4
  In5 : Inport  Port=5
  In6 : Inport  Port=6
  In7 : Inport  Port=7
  NAND : Logic  Operator=NAND  AllPortsSameDT=off  OutDataTypeStr=boolean
  NAND{1..2,4..6} (5 alike) : Logic  Operator=NAND  Inputs=4  AllPortsSameDT=off  OutDataTypeStr=boolean
  NAND3 : Logic  Operator=NAND  AllPortsSameDT=off  OutDataTypeStr=boolean
  Out1 : Outport
  wires:
  NAND6/1 -> NAND1/4
  In5/1 -> NAND5/3
  NAND3/1 -> NAND4/2, NAND2/2
  In1/1 -> NAND6/2, NAND5/2, NAND3/2, NAND3/1
  In2/1 -> NAND6/1, NAND4/1, NAND/2, NAND/1
  In4/1 -> NAND4/3
  In3/1 -> NAND2/3
  NAND/1 -> NAND5/1, NAND2/1
  NAND1/1 -> Out1/1
  In6/1 -> NAND6/3
  NAND5/1 -> NAND1/3
  NAND4/1 -> NAND1/2
  In7/1 -> NAND2/4, NAND4/4, NAND5/4, NAND6/4
  NAND2/1 -> NAND1/1

== system bit32cpu/ALU/Subsystem7/Subsystem4/Subsystem3/Subsystem5 ==
  In1 : Inport
  In2 : Inport  Port=2
  In3 : Inport  Port=3
  In4 : Inport  Port=4
  In5 : Inport  Port=5
  In6 : Inport  Port=6
  In7 : Inport  Port=7
  NAND : Logic  Operator=NAND  AllPortsSameDT=off  OutDataTypeStr=boolean
  NAND{1..2,4..6} (5 alike) : Logic  Operator=NAND  Inputs=4  AllPortsSameDT=off  OutDataTypeStr=boolean
  NAND3 : Logic  Operator=NAND  AllPortsSameDT=off  OutDataTypeStr=boolean
  Out1 : Outport
  wires:
  NAND6/1 -> NAND1/4
  In5/1 -> NAND5/3
  NAND3/1 -> NAND4/2, NAND2/2
  In1/1 -> NAND6/2, NAND5/2, NAND3/2, NAND3/1
  In2/1 -> NAND6/1, NAND4/1, NAND/2, NAND/1
  In4/1 -> NAND4/3
  In3/1 -> NAND2/3
  NAND/1 -> NAND5/1, NAND2/1
  NAND1/1 -> Out1/1
  In6/1 -> NAND6/3
  NAND5/1 -> NAND1/3
  NAND4/1 -> NAND1/2
  In7/1 -> NAND2/4, NAND4/4, NAND5/4, NAND6/4
  NAND2/1 -> NAND1/1

== system bit32cpu/ALU/Subsystem7/Subsystem4/Subsystem3/Subsystem6 ==
  In1 : Inport
  In2 : Inport  Port=2
  In3 : Inport  Port=3
  In4 : Inport  Port=4
  In5 : Inport  Port=5
  In6 : Inport  Port=6
  In7 : Inport  Port=7
  NAND : Logic  Operator=NAND  AllPortsSameDT=off  OutDataTypeStr=boolean
  NAND{1..2,4..6} (5 alike) : Logic  Operator=NAND  Inputs=4  AllPortsSameDT=off  OutDataTypeStr=boolean
  NAND3 : Logic  Operator=NAND  AllPortsSameDT=off  OutDataTypeStr=boolean
  Out1 : Outport
  wires:
  NAND6/1 -> NAND1/4
  In5/1 -> NAND5/3
  NAND3/1 -> NAND4/2, NAND2/2
  In1/1 -> NAND6/2, NAND5/2, NAND3/2, NAND3/1
  In2/1 -> NAND6/1, NAND4/1, NAND/2, NAND/1
  In4/1 -> NAND4/3
  In3/1 -> NAND2/3
  NAND/1 -> NAND5/1, NAND2/1
  NAND1/1 -> Out1/1
  In6/1 -> NAND6/3
  NAND5/1 -> NAND1/3
  NAND4/1 -> NAND1/2
  In7/1 -> NAND2/4, NAND4/4, NAND5/4, NAND6/4
  NAND2/1 -> NAND1/1

== system bit32cpu/ALU/Subsystem7/Subsystem4/Subsystem3/Subsystem7 ==
  In1 : Inport
  In2 : Inport  Port=2
  In3 : Inport  Port=3
  In4 : Inport  Port=4
  In5 : Inport  Port=5
  In6 : Inport  Port=6
  In7 : Inport  Port=7
  NAND : Logic  Operator=NAND  AllPortsSameDT=off  OutDataTypeStr=boolean
  NAND{1..2,4..6} (5 alike) : Logic  Operator=NAND  Inputs=4  AllPortsSameDT=off  OutDataTypeStr=boolean
  NAND3 : Logic  Operator=NAND  AllPortsSameDT=off  OutDataTypeStr=boolean
  Out1 : Outport
  wires:
  NAND6/1 -> NAND1/4
  In5/1 -> NAND5/3
  NAND3/1 -> NAND4/2, NAND2/2
  In1/1 -> NAND6/2, NAND5/2, NAND3/2, NAND3/1
  In2/1 -> NAND6/1, NAND4/1, NAND/2, NAND/1
  In4/1 -> NAND4/3
  In3/1 -> NAND2/3
  NAND/1 -> NAND5/1, NAND2/1
  NAND1/1 -> Out1/1
  In6/1 -> NAND6/3
  NAND5/1 -> NAND1/3
  NAND4/1 -> NAND1/2
  In7/1 -> NAND2/4, NAND4/4, NAND5/4, NAND6/4
  NAND2/1 -> NAND1/1

== system bit32cpu/ALU/Subsystem7/Subsystem4/Subsystem4/Subsystem ==
  In1 : Inport
  In2 : Inport  Port=2
  In3 : Inport  Port=3
  In4 : Inport  Port=4
  In5 : Inport  Port=5
  In6 : Inport  Port=6
  In7 : Inport  Port=7
  NAND : Logic  Operator=NAND  AllPortsSameDT=off  OutDataTypeStr=boolean
  NAND{1..2,4..6} (5 alike) : Logic  Operator=NAND  Inputs=4  AllPortsSameDT=off  OutDataTypeStr=boolean
  NAND3 : Logic  Operator=NAND  AllPortsSameDT=off  OutDataTypeStr=boolean
  Out1 : Outport
  wires:
  NAND6/1 -> NAND1/4
  In5/1 -> NAND5/3
  NAND3/1 -> NAND4/2, NAND2/2
  In1/1 -> NAND6/2, NAND5/2, NAND3/2, NAND3/1
  In2/1 -> NAND6/1, NAND4/1, NAND/2, NAND/1
  In4/1 -> NAND4/3
  In3/1 -> NAND2/3
  NAND/1 -> NAND5/1, NAND2/1
  NAND1/1 -> Out1/1
  In6/1 -> NAND6/3
  NAND5/1 -> NAND1/3
  NAND4/1 -> NAND1/2
  In7/1 -> NAND2/4, NAND4/4, NAND5/4, NAND6/4
  NAND2/1 -> NAND1/1

== system bit32cpu/ALU/Subsystem7/Subsystem4/Subsystem4/Subsystem1 ==
  In1 : Inport
  In2 : Inport  Port=2
  In3 : Inport  Port=3
  In4 : Inport  Port=4
  In5 : Inport  Port=5
  In6 : Inport  Port=6
  In7 : Inport  Port=7
  NAND : Logic  Operator=NAND  AllPortsSameDT=off  OutDataTypeStr=boolean
  NAND{1..2,4..6} (5 alike) : Logic  Operator=NAND  Inputs=4  AllPortsSameDT=off  OutDataTypeStr=boolean
  NAND3 : Logic  Operator=NAND  AllPortsSameDT=off  OutDataTypeStr=boolean
  Out1 : Outport
  wires:
  NAND6/1 -> NAND1/4
  In5/1 -> NAND5/3
  NAND3/1 -> NAND4/2, NAND2/2
  In1/1 -> NAND6/2, NAND5/2, NAND3/2, NAND3/1
  In2/1 -> NAND6/1, NAND4/1, NAND/2, NAND/1
  In4/1 -> NAND4/3
  In3/1 -> NAND2/3
  NAND/1 -> NAND5/1, NAND2/1
  NAND1/1 -> Out1/1
  In6/1 -> NAND6/3
  NAND5/1 -> NAND1/3
  NAND4/1 -> NAND1/2
  In7/1 -> NAND2/4, NAND4/4, NAND5/4, NAND6/4
  NAND2/1 -> NAND1/1

== system bit32cpu/ALU/Subsystem7/Subsystem4/Subsystem4/Subsystem2 ==
  In1 : Inport
  In2 : Inport  Port=2
  In3 : Inport  Port=3
  In4 : Inport  Port=4
  In5 : Inport  Port=5
  In6 : Inport  Port=6
  In7 : Inport  Port=7
  NAND : Logic  Operator=NAND  AllPortsSameDT=off  OutDataTypeStr=boolean
  NAND{1..2,4..6} (5 alike) : Logic  Operator=NAND  Inputs=4  AllPortsSameDT=off  OutDataTypeStr=boolean
  NAND3 : Logic  Operator=NAND  AllPortsSameDT=off  OutDataTypeStr=boolean
  Out1 : Outport
  wires:
  NAND6/1 -> NAND1/4
  In5/1 -> NAND5/3
  NAND3/1 -> NAND4/2, NAND2/2
  In1/1 -> NAND6/2, NAND5/2, NAND3/2, NAND3/1
  In2/1 -> NAND6/1, NAND4/1, NAND/2, NAND/1
  In4/1 -> NAND4/3
  In3/1 -> NAND2/3
  NAND/1 -> NAND5/1, NAND2/1
  NAND1/1 -> Out1/1
  In6/1 -> NAND6/3
  NAND5/1 -> NAND1/3
  NAND4/1 -> NAND1/2
  In7/1 -> NAND2/4, NAND4/4, NAND5/4, NAND6/4
  NAND2/1 -> NAND1/1

== system bit32cpu/ALU/Subsystem7/Subsystem4/Subsystem4/Subsystem3 ==
  In1 : Inport
  In2 : Inport  Port=2
  In3 : Inport  Port=3
  In4 : Inport  Port=4
  In5 : Inport  Port=5
  In6 : Inport  Port=6
  In7 : Inport  Port=7
  NAND : Logic  Operator=NAND  AllPortsSameDT=off  OutDataTypeStr=boolean
  NAND{1..2,4..6} (5 alike) : Logic  Operator=NAND  Inputs=4  AllPortsSameDT=off  OutDataTypeStr=boolean
  NAND3 : Logic  Operator=NAND  AllPortsSameDT=off  OutDataTypeStr=boolean
  Out1 : Outport
  wires:
  NAND6/1 -> NAND1/4
  In5/1 -> NAND5/3
  NAND3/1 -> NAND4/2, NAND2/2
  In1/1 -> NAND6/2, NAND5/2, NAND3/2, NAND3/1
  In2/1 -> NAND6/1, NAND4/1, NAND/2, NAND/1
  In4/1 -> NAND4/3
  In3/1 -> NAND2/3
  NAND/1 -> NAND5/1, NAND2/1
  NAND1/1 -> Out1/1
  In6/1 -> NAND6/3
  NAND5/1 -> NAND1/3
  NAND4/1 -> NAND1/2
  In7/1 -> NAND2/4, NAND4/4, NAND5/4, NAND6/4
  NAND2/1 -> NAND1/1

== system bit32cpu/ALU/Subsystem7/Subsystem4/Subsystem4/Subsystem4 ==
  In1 : Inport
  In2 : Inport  Port=2
  In3 : Inport  Port=3
  In4 : Inport  Port=4
  In5 : Inport  Port=5
  In6 : Inport  Port=6
  In7 : Inport  Port=7
  NAND : Logic  Operator=NAND  AllPortsSameDT=off  OutDataTypeStr=boolean
  NAND{1..2,4..6} (5 alike) : Logic  Operator=NAND  Inputs=4  AllPortsSameDT=off  OutDataTypeStr=boolean
  NAND3 : Logic  Operator=NAND  AllPortsSameDT=off  OutDataTypeStr=boolean
  Out1 : Outport
  wires:
  NAND6/1 -> NAND1/4
  In5/1 -> NAND5/3
  NAND3/1 -> NAND4/2, NAND2/2
  In1/1 -> NAND6/2, NAND5/2, NAND3/2, NAND3/1
  In2/1 -> NAND6/1, NAND4/1, NAND/2, NAND/1
  In4/1 -> NAND4/3
  In3/1 -> NAND2/3
  NAND/1 -> NAND5/1, NAND2/1
  NAND1/1 -> Out1/1
  In6/1 -> NAND6/3
  NAND5/1 -> NAND1/3
  NAND4/1 -> NAND1/2
  In7/1 -> NAND2/4, NAND4/4, NAND5/4, NAND6/4
  NAND2/1 -> NAND1/1

== system bit32cpu/ALU/Subsystem7/Subsystem4/Subsystem4/Subsystem5 ==
  In1 : Inport
  In2 : Inport  Port=2
  In3 : Inport  Port=3
  In4 : Inport  Port=4
  In5 : Inport  Port=5
  In6 : Inport  Port=6
  In7 : Inport  Port=7
  NAND : Logic  Operator=NAND  AllPortsSameDT=off  OutDataTypeStr=boolean
  NAND{1..2,4..6} (5 alike) : Logic  Operator=NAND  Inputs=4  AllPortsSameDT=off  OutDataTypeStr=boolean
  NAND3 : Logic  Operator=NAND  AllPortsSameDT=off  OutDataTypeStr=boolean
  Out1 : Outport
  wires:
  NAND6/1 -> NAND1/4
  In5/1 -> NAND5/3
  NAND3/1 -> NAND4/2, NAND2/2
  In1/1 -> NAND6/2, NAND5/2, NAND3/2, NAND3/1
  In2/1 -> NAND6/1, NAND4/1, NAND/2, NAND/1
  In4/1 -> NAND4/3
  In3/1 -> NAND2/3
  NAND/1 -> NAND5/1, NAND2/1
  NAND1/1 -> Out1/1
  In6/1 -> NAND6/3
  NAND5/1 -> NAND1/3
  NAND4/1 -> NAND1/2
  In7/1 -> NAND2/4, NAND4/4, NAND5/4, NAND6/4
  NAND2/1 -> NAND1/1

== system bit32cpu/ALU/Subsystem7/Subsystem4/Subsystem4/Subsystem6 ==
  In1 : Inport
  In2 : Inport  Port=2
  In3 : Inport  Port=3
  In4 : Inport  Port=4
  In5 : Inport  Port=5
  In6 : Inport  Port=6
  In7 : Inport  Port=7
  NAND : Logic  Operator=NAND  AllPortsSameDT=off  OutDataTypeStr=boolean
  NAND{1..2,4..6} (5 alike) : Logic  Operator=NAND  Inputs=4  AllPortsSameDT=off  OutDataTypeStr=boolean
  NAND3 : Logic  Operator=NAND  AllPortsSameDT=off  OutDataTypeStr=boolean
  Out1 : Outport
  wires:
  NAND6/1 -> NAND1/4
  In5/1 -> NAND5/3
  NAND3/1 -> NAND4/2, NAND2/2
  In1/1 -> NAND6/2, NAND5/2, NAND3/2, NAND3/1
  In2/1 -> NAND6/1, NAND4/1, NAND/2, NAND/1
  In4/1 -> NAND4/3
  In3/1 -> NAND2/3
  NAND/1 -> NAND5/1, NAND2/1
  NAND1/1 -> Out1/1
  In6/1 -> NAND6/3
  NAND5/1 -> NAND1/3
  NAND4/1 -> NAND1/2
  In7/1 -> NAND2/4, NAND4/4, NAND5/4, NAND6/4
  NAND2/1 -> NAND1/1

== system bit32cpu/ALU/Subsystem7/Subsystem4/Subsystem4/Subsystem7 ==
  In1 : Inport
  In2 : Inport  Port=2
  In3 : Inport  Port=3
  In4 : Inport  Port=4
  In5 : Inport  Port=5
  In6 : Inport  Port=6
  In7 : Inport  Port=7
  NAND : Logic  Operator=NAND  AllPortsSameDT=off  OutDataTypeStr=boolean
  NAND{1..2,4..6} (5 alike) : Logic  Operator=NAND  Inputs=4  AllPortsSameDT=off  OutDataTypeStr=boolean
  NAND3 : Logic  Operator=NAND  AllPortsSameDT=off  OutDataTypeStr=boolean
  Out1 : Outport
  wires:
  NAND6/1 -> NAND1/4
  In5/1 -> NAND5/3
  NAND3/1 -> NAND4/2, NAND2/2
  In1/1 -> NAND6/2, NAND5/2, NAND3/2, NAND3/1
  In2/1 -> NAND6/1, NAND4/1, NAND/2, NAND/1
  In4/1 -> NAND4/3
  In3/1 -> NAND2/3
  NAND/1 -> NAND5/1, NAND2/1
  NAND1/1 -> Out1/1
  In6/1 -> NAND6/3
  NAND5/1 -> NAND1/3
  NAND4/1 -> NAND1/2
  In7/1 -> NAND2/4, NAND4/4, NAND5/4, NAND6/4
  NAND2/1 -> NAND1/1

== system bit32cpu/ALU/Subsystem7/Subsystem4/Subsystem5/Subsystem ==
  In1 : Inport
  In2 : Inport  Port=2
  In3 : Inport  Port=3
  In4 : Inport  Port=4
  In5 : Inport  Port=5
  In6 : Inport  Port=6
  In7 : Inport  Port=7
  NAND : Logic  Operator=NAND  AllPortsSameDT=off  OutDataTypeStr=boolean
  NAND{1..2,4..6} (5 alike) : Logic  Operator=NAND  Inputs=4  AllPortsSameDT=off  OutDataTypeStr=boolean
  NAND3 : Logic  Operator=NAND  AllPortsSameDT=off  OutDataTypeStr=boolean
  Out1 : Outport
  wires:
  NAND6/1 -> NAND1/4
  In5/1 -> NAND5/3
  NAND3/1 -> NAND4/2, NAND2/2
  In1/1 -> NAND6/2, NAND5/2, NAND3/2, NAND3/1
  In2/1 -> NAND6/1, NAND4/1, NAND/2, NAND/1
  In4/1 -> NAND4/3
  In3/1 -> NAND2/3
  NAND/1 -> NAND5/1, NAND2/1
  NAND1/1 -> Out1/1
  In6/1 -> NAND6/3
  NAND5/1 -> NAND1/3
  NAND4/1 -> NAND1/2
  In7/1 -> NAND2/4, NAND4/4, NAND5/4, NAND6/4
  NAND2/1 -> NAND1/1

== system bit32cpu/ALU/Subsystem7/Subsystem4/Subsystem5/Subsystem1 ==
  In1 : Inport
  In2 : Inport  Port=2
  In3 : Inport  Port=3
  In4 : Inport  Port=4
  In5 : Inport  Port=5
  In6 : Inport  Port=6
  In7 : Inport  Port=7
  NAND : Logic  Operator=NAND  AllPortsSameDT=off  OutDataTypeStr=boolean
  NAND{1..2,4..6} (5 alike) : Logic  Operator=NAND  Inputs=4  AllPortsSameDT=off  OutDataTypeStr=boolean
  NAND3 : Logic  Operator=NAND  AllPortsSameDT=off  OutDataTypeStr=boolean
  Out1 : Outport
  wires:
  NAND6/1 -> NAND1/4
  In5/1 -> NAND5/3
  NAND3/1 -> NAND4/2, NAND2/2
  In1/1 -> NAND6/2, NAND5/2, NAND3/2, NAND3/1
  In2/1 -> NAND6/1, NAND4/1, NAND/2, NAND/1
  In4/1 -> NAND4/3
  In3/1 -> NAND2/3
  NAND/1 -> NAND5/1, NAND2/1
  NAND1/1 -> Out1/1
  In6/1 -> NAND6/3
  NAND5/1 -> NAND1/3
  NAND4/1 -> NAND1/2
  In7/1 -> NAND2/4, NAND4/4, NAND5/4, NAND6/4
  NAND2/1 -> NAND1/1

== system bit32cpu/ALU/Subsystem7/Subsystem4/Subsystem5/Subsystem2 ==
  In1 : Inport
  In2 : Inport  Port=2
  In3 : Inport  Port=3
  In4 : Inport  Port=4
  In5 : Inport  Port=5
  In6 : Inport  Port=6
  In7 : Inport  Port=7
  NAND : Logic  Operator=NAND  AllPortsSameDT=off  OutDataTypeStr=boolean
  NAND{1..2,4..6} (5 alike) : Logic  Operator=NAND  Inputs=4  AllPortsSameDT=off  OutDataTypeStr=boolean
  NAND3 : Logic  Operator=NAND  AllPortsSameDT=off  OutDataTypeStr=boolean
  Out1 : Outport
  wires:
  NAND6/1 -> NAND1/4
  In5/1 -> NAND5/3
  NAND3/1 -> NAND4/2, NAND2/2
  In1/1 -> NAND6/2, NAND5/2, NAND3/2, NAND3/1
  In2/1 -> NAND6/1, NAND4/1, NAND/2, NAND/1
  In4/1 -> NAND4/3
  In3/1 -> NAND2/3
  NAND/1 -> NAND5/1, NAND2/1
  NAND1/1 -> Out1/1
  In6/1 -> NAND6/3
  NAND5/1 -> NAND1/3
  NAND4/1 -> NAND1/2
  In7/1 -> NAND2/4, NAND4/4, NAND5/4, NAND6/4
  NAND2/1 -> NAND1/1

== system bit32cpu/ALU/Subsystem7/Subsystem4/Subsystem5/Subsystem3 ==
  In1 : Inport
  In2 : Inport  Port=2
  In3 : Inport  Port=3
  In4 : Inport  Port=4
  In5 : Inport  Port=5
  In6 : Inport  Port=6
  In7 : Inport  Port=7
  NAND : Logic  Operator=NAND  AllPortsSameDT=off  OutDataTypeStr=boolean
  NAND{1..2,4..6} (5 alike) : Logic  Operator=NAND  Inputs=4  AllPortsSameDT=off  OutDataTypeStr=boolean
  NAND3 : Logic  Operator=NAND  AllPortsSameDT=off  OutDataTypeStr=boolean
  Out1 : Outport
  wires:
  NAND6/1 -> NAND1/4
  In5/1 -> NAND5/3
  NAND3/1 -> NAND4/2, NAND2/2
  In1/1 -> NAND6/2, NAND5/2, NAND3/2, NAND3/1
  In2/1 -> NAND6/1, NAND4/1, NAND/2, NAND/1
  In4/1 -> NAND4/3
  In3/1 -> NAND2/3
  NAND/1 -> NAND5/1, NAND2/1
  NAND1/1 -> Out1/1
  In6/1 -> NAND6/3
  NAND5/1 -> NAND1/3
  NAND4/1 -> NAND1/2
  In7/1 -> NAND2/4, NAND4/4, NAND5/4, NAND6/4
  NAND2/1 -> NAND1/1

== system bit32cpu/ALU/Subsystem7/Subsystem4/Subsystem5/Subsystem4 ==
  In1 : Inport
  In2 : Inport  Port=2
  In3 : Inport  Port=3
  In4 : Inport  Port=4
  In5 : Inport  Port=5
  In6 : Inport  Port=6
  In7 : Inport  Port=7
  NAND : Logic  Operator=NAND  AllPortsSameDT=off  OutDataTypeStr=boolean
  NAND{1..2,4..6} (5 alike) : Logic  Operator=NAND  Inputs=4  AllPortsSameDT=off  OutDataTypeStr=boolean
  NAND3 : Logic  Operator=NAND  AllPortsSameDT=off  OutDataTypeStr=boolean
  Out1 : Outport
  wires:
  NAND6/1 -> NAND1/4
  In5/1 -> NAND5/3
  NAND3/1 -> NAND4/2, NAND2/2
  In1/1 -> NAND6/2, NAND5/2, NAND3/2, NAND3/1
  In2/1 -> NAND6/1, NAND4/1, NAND/2, NAND/1
  In4/1 -> NAND4/3
  In3/1 -> NAND2/3
  NAND/1 -> NAND5/1, NAND2/1
  NAND1/1 -> Out1/1
  In6/1 -> NAND6/3
  NAND5/1 -> NAND1/3
  NAND4/1 -> NAND1/2
  In7/1 -> NAND2/4, NAND4/4, NAND5/4, NAND6/4
  NAND2/1 -> NAND1/1

== system bit32cpu/ALU/Subsystem7/Subsystem4/Subsystem5/Subsystem5 ==
  In1 : Inport
  In2 : Inport  Port=2
  In3 : Inport  Port=3
  In4 : Inport  Port=4
  In5 : Inport  Port=5
  In6 : Inport  Port=6
  In7 : Inport  Port=7
  NAND : Logic  Operator=NAND  AllPortsSameDT=off  OutDataTypeStr=boolean
  NAND{1..2,4..6} (5 alike) : Logic  Operator=NAND  Inputs=4  AllPortsSameDT=off  OutDataTypeStr=boolean
  NAND3 : Logic  Operator=NAND  AllPortsSameDT=off  OutDataTypeStr=boolean
  Out1 : Outport
  wires:
  NAND6/1 -> NAND1/4
  In5/1 -> NAND5/3
  NAND3/1 -> NAND4/2, NAND2/2
  In1/1 -> NAND6/2, NAND5/2, NAND3/2, NAND3/1
  In2/1 -> NAND6/1, NAND4/1, NAND/2, NAND/1
  In4/1 -> NAND4/3
  In3/1 -> NAND2/3
  NAND/1 -> NAND5/1, NAND2/1
  NAND1/1 -> Out1/1
  In6/1 -> NAND6/3
  NAND5/1 -> NAND1/3
  NAND4/1 -> NAND1/2
  In7/1 -> NAND2/4, NAND4/4, NAND5/4, NAND6/4
  NAND2/1 -> NAND1/1

== system bit32cpu/ALU/Subsystem7/Subsystem4/Subsystem5/Subsystem6 ==
  In1 : Inport
  In2 : Inport  Port=2
  In3 : Inport  Port=3
  In4 : Inport  Port=4
  In5 : Inport  Port=5
  In6 : Inport  Port=6
  In7 : Inport  Port=7
  NAND : Logic  Operator=NAND  AllPortsSameDT=off  OutDataTypeStr=boolean
  NAND{1..2,4..6} (5 alike) : Logic  Operator=NAND  Inputs=4  AllPortsSameDT=off  OutDataTypeStr=boolean
  NAND3 : Logic  Operator=NAND  AllPortsSameDT=off  OutDataTypeStr=boolean
  Out1 : Outport
  wires:
  NAND6/1 -> NAND1/4
  In5/1 -> NAND5/3
  NAND3/1 -> NAND4/2, NAND2/2
  In1/1 -> NAND6/2, NAND5/2, NAND3/2, NAND3/1
  In2/1 -> NAND6/1, NAND4/1, NAND/2, NAND/1
  In4/1 -> NAND4/3
  In3/1 -> NAND2/3
  NAND/1 -> NAND5/1, NAND2/1
  NAND1/1 -> Out1/1
  In6/1 -> NAND6/3
  NAND5/1 -> NAND1/3
  NAND4/1 -> NAND1/2
  In7/1 -> NAND2/4, NAND4/4, NAND5/4, NAND6/4
  NAND2/1 -> NAND1/1

== system bit32cpu/ALU/Subsystem7/Subsystem4/Subsystem5/Subsystem7 ==
  In1 : Inport
  In2 : Inport  Port=2
  In3 : Inport  Port=3
  In4 : Inport  Port=4
  In5 : Inport  Port=5
  In6 : Inport  Port=6
  In7 : Inport  Port=7
  NAND : Logic  Operator=NAND  AllPortsSameDT=off  OutDataTypeStr=boolean
  NAND{1..2,4..6} (5 alike) : Logic  Operator=NAND  Inputs=4  AllPortsSameDT=off  OutDataTypeStr=boolean
  NAND3 : Logic  Operator=NAND  AllPortsSameDT=off  OutDataTypeStr=boolean
  Out1 : Outport
  wires:
  NAND6/1 -> NAND1/4
  In5/1 -> NAND5/3
  NAND3/1 -> NAND4/2, NAND2/2
  In1/1 -> NAND6/2, NAND5/2, NAND3/2, NAND3/1
  In2/1 -> NAND6/1, NAND4/1, NAND/2, NAND/1
  In4/1 -> NAND4/3
  In3/1 -> NAND2/3
  NAND/1 -> NAND5/1, NAND2/1
  NAND1/1 -> Out1/1
  In6/1 -> NAND6/3
  NAND5/1 -> NAND1/3
  NAND4/1 -> NAND1/2
  In7/1 -> NAND2/4, NAND4/4, NAND5/4, NAND6/4
  NAND2/1 -> NAND1/1

== system bit32cpu/ALU/Subtractor/Subtractor/Subsystem1/Subsystem ==
  In1 : Inport
  In2 : Inport  Port=2
  In3 : Inport  Port=3
  Demux : Demux  Outputs=2
  Demux1 : Demux  Outputs=2
  Mux : Mux  Inputs=2
  Subsystem1 : Subsystem
  Subsystem2 : Subsystem
  Out1 : Outport
  Out2 : Outport  Port=2
  wires:
  Subsystem2/1(Out1) -> Out1/1
  In3/1 -> Demux1/1
  Demux/1 -> Subsystem2/1(In1)
  Subsystem1/1(Out1) -> Subsystem2/2(In2)
  In2/1 -> Subsystem1/2(In2)
  In1/1 -> Demux/1
  Demux1/1 -> Subsystem2/3(In3)
  Mux/1 -> Out2/1
  Demux1/2 -> Subsystem1/3(In3)
  Demux/2 -> Subsystem1/1(In1)
  Subsystem2/2(Out2) -> Mux/1
  Subsystem1/2(Out2) -> Mux/2

== system bit32cpu/ALU/Subtractor/Subtractor/Subsystem1/Subsystem1 ==
  In1 : Inport
  In2 : Inport  Port=2
  In3 : Inport  Port=3
  Demux : Demux  Outputs=2
  Demux1 : Demux  Outputs=2
  Mux : Mux  Inputs=2
  Subsystem1 : Subsystem
  Subsystem2 : Subsystem
  Out1 : Outport
  Out2 : Outport  Port=2
  wires:
  Subsystem2/1(Out1) -> Out1/1
  In3/1 -> Demux1/1
  Demux/1 -> Subsystem2/1(In1)
  Subsystem1/1(Out1) -> Subsystem2/2(In2)
  In2/1 -> Subsystem1/2(In2)
  In1/1 -> Demux/1
  Demux1/1 -> Subsystem2/3(In3)
  Mux/1 -> Out2/1
  Demux1/2 -> Subsystem1/3(In3)
  Demux/2 -> Subsystem1/1(In1)
  Subsystem2/2(Out2) -> Mux/1
  Subsystem1/2(Out2) -> Mux/2

== system bit32cpu/ALU/Subtractor/Subtractor/Subsystem2/Subsystem ==
  In1 : Inport
  In2 : Inport  Port=2
  In3 : Inport  Port=3
  Demux : Demux  Outputs=2
  Demux1 : Demux  Outputs=2
  Mux : Mux  Inputs=2
  Subsystem1 : Subsystem
  Subsystem2 : Subsystem
  Out1 : Outport
  Out2 : Outport  Port=2
  wires:
  Subsystem2/1(Out1) -> Out1/1
  In3/1 -> Demux1/1
  Demux/1 -> Subsystem2/1(In1)
  Subsystem1/1(Out1) -> Subsystem2/2(In2)
  In2/1 -> Subsystem1/2(In2)
  In1/1 -> Demux/1
  Demux1/1 -> Subsystem2/3(In3)
  Mux/1 -> Out2/1
  Demux1/2 -> Subsystem1/3(In3)
  Demux/2 -> Subsystem1/1(In1)
  Subsystem2/2(Out2) -> Mux/1
  Subsystem1/2(Out2) -> Mux/2

== system bit32cpu/ALU/Subtractor/Subtractor/Subsystem2/Subsystem1 ==
  In1 : Inport
  In2 : Inport  Port=2
  In3 : Inport  Port=3
  Demux : Demux  Outputs=2
  Demux1 : Demux  Outputs=2
  Mux : Mux  Inputs=2
  Subsystem1 : Subsystem
  Subsystem2 : Subsystem
  Out1 : Outport
  Out2 : Outport  Port=2
  wires:
  Subsystem2/1(Out1) -> Out1/1
  In3/1 -> Demux1/1
  Demux/1 -> Subsystem2/1(In1)
  Subsystem1/1(Out1) -> Subsystem2/2(In2)
  In2/1 -> Subsystem1/2(In2)
  In1/1 -> Demux/1
  Demux1/1 -> Subsystem2/3(In3)
  Mux/1 -> Out2/1
  Demux1/2 -> Subsystem1/3(In3)
  Demux/2 -> Subsystem1/1(In1)
  Subsystem2/2(Out2) -> Mux/1
  Subsystem1/2(Out2) -> Mux/2

== system bit32cpu/ALU/Adder/Subsystem/Subsystem1/Subsystem/Subsystem1 ==
  In1 : Inport
  In2 : Inport  Port=2
  In3 : Inport  Port=3
  Demux : Demux
  Demux1 : Demux
  Mux : Mux
  Subsystem : Subsystem
  Out1 : Outport
  Out2 : Outport  Port=2
  wires:
  Demux/1 -> Subsystem/1(In1)
  Subsystem/4(Out4) -> Mux/3
  Demux/4 -> Subsystem/4(In4)
  Subsystem/3(Out3) -> Mux/2
  Subsystem/2(Out2) -> Mux/1
  In2/1 -> Subsystem/5(In5)
  Mux/1 -> Out2/1
  In3/1 -> Demux1/1
  Demux1/1 -> Subsystem/6(In6)
  Demux1/2 -> Subsystem/7(In7)
  Demux/2 -> Subsystem/2(In2)
  In1/1 -> Demux/1
  Subsystem/1(Out1) -> Out1/1
  Subsystem/5(Out5) -> Mux/4
  Demux1/3 -> Subsystem/8(In8)
  Demux1/4 -> Subsystem/9(In9)
  Demux/3 -> Subsystem/3(In3)

== system bit32cpu/ALU/Adder/Subsystem/Subsystem1/Subsystem/Subsystem2 ==
  In1 : Inport
  In2 : Inport  Port=2
  In3 : Inport  Port=3
  Demux : Demux
  Demux1 : Demux
  Mux : Mux
  Subsystem : Subsystem
  Out1 : Outport
  Out2 : Outport  Port=2
  wires:
  Demux/1 -> Subsystem/1(In1)
  Subsystem/4(Out4) -> Mux/3
  Demux/4 -> Subsystem/4(In4)
  Subsystem/3(Out3) -> Mux/2
  Subsystem/2(Out2) -> Mux/1
  In2/1 -> Subsystem/5(In5)
  Mux/1 -> Out2/1
  In3/1 -> Demux1/1
  Demux1/1 -> Subsystem/6(In6)
  Demux1/2 -> Subsystem/7(In7)
  Demux/2 -> Subsystem/2(In2)
  In1/1 -> Demux/1
  Subsystem/1(Out1) -> Out1/1
  Subsystem/5(Out5) -> Mux/4
  Demux1/3 -> Subsystem/8(In8)
  Demux1/4 -> Subsystem/9(In9)
  Demux/3 -> Subsystem/3(In3)

== system bit32cpu/ALU/Adder/Subsystem/Subsystem1/Subsystem1/Subsystem1 ==
  In1 : Inport
  In2 : Inport  Port=2
  In3 : Inport  Port=3
  Demux : Demux
  Demux1 : Demux
  Mux : Mux
  Subsystem : Subsystem
  Out1 : Outport
  Out2 : Outport  Port=2
  wires:
  Demux/1 -> Subsystem/1(In1)
  Subsystem/4(Out4) -> Mux/3
  Demux/4 -> Subsystem/4(In4)
  Subsystem/3(Out3) -> Mux/2
  Subsystem/2(Out2) -> Mux/1
  In2/1 -> Subsystem/5(In5)
  Mux/1 -> Out2/1
  In3/1 -> Demux1/1
  Demux1/1 -> Subsystem/6(In6)
  Demux1/2 -> Subsystem/7(In7)
  Demux/2 -> Subsystem/2(In2)
  In1/1 -> Demux/1
  Subsystem/1(Out1) -> Out1/1
  Subsystem/5(Out5) -> Mux/4
  Demux1/3 -> Subsystem/8(In8)
  Demux1/4 -> Subsystem/9(In9)
  Demux/3 -> Subsystem/3(In3)
